simulink model "DETM"  (R2018b)
settings: Solver=ode3  StartTime=0.0  StopTime=55  FixedStep=0.0008  RelTol=1e-3
settings Model: Creator=SURFACE  LastModifiedBy=SURFACE

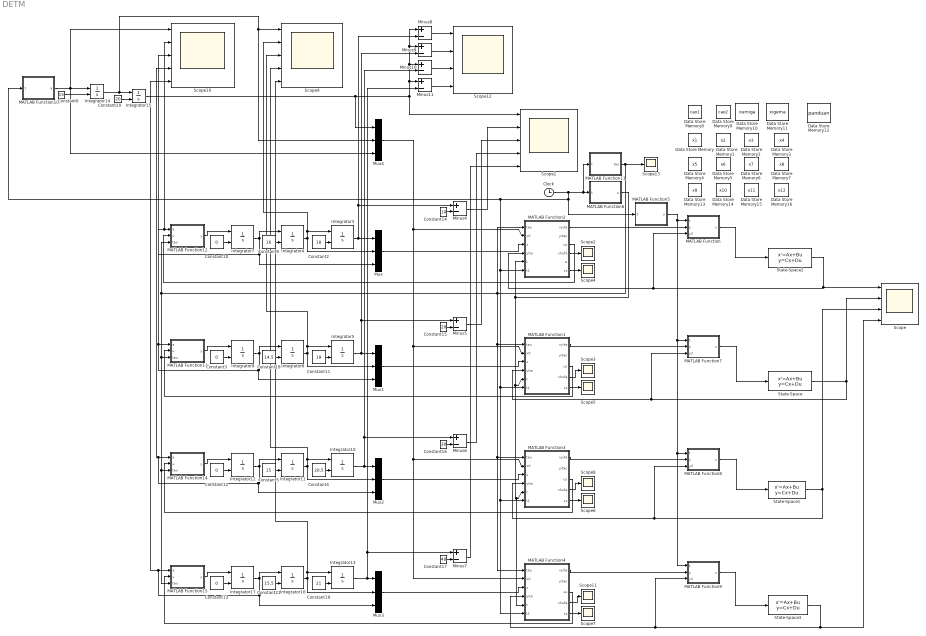
== system DETM ==
  Clock : Clock
  Constant{3,10,12..13} (4 alike) : Constant  Value=0
  Constant11 : Constant  Value=19
  Constant14 : Constant  Value=10
  Constant15 : Constant  Value=20
  Constant16 : Constant  Value=30
  Constant17 : Constant  Value=40
  Constant18 : Constant  Value=14.5
  Constant19 : Constant  Value=21
  Constant2 : Constant  Value=18
  Constant20 : Constant  Value=20
  Constant21 : Constant  Value=15.5
  Constant4 : Constant  Value=20.5
  Constant5 : Constant  Value=15
  Constant6 : Constant  Value=15
  Constant9 : Constant  Value=16
  Data Store Memory : DataStoreMemory  DataStoreName=x1  ReadBeforeWriteMsg=warning  WriteAfterWriteMsg=warning  WriteAfterReadMsg=warning  InitialValue=[18;16;0]  ShowAdditionalParam=off  OutDataTypeStr=double  Dimensions=3
  Data Store Memory1 : DataStoreMemory  DataStoreName=x2  ReadBeforeWriteMsg=warning  WriteAfterWriteMsg=warning  WriteAfterReadMsg=warning  InitialValue=[19;14.5;0]  ShowAdditionalParam=off  OutDataTypeStr=double  Dimensions=3
  Data Store Memory10 : DataStoreMemory  DataStoreName=oumiga  ReadBeforeWriteMsg=warning  WriteAfterWriteMsg=warning  WriteAfterReadMsg=warning  InitialValue=0.5  ShowAdditionalParam=off  OutDataTypeStr=double  Dimensions=1
  Data Store Memory11 : DataStoreMemory  DataStoreName=xigema  ReadBeforeWriteMsg=warning  WriteAfterWriteMsg=warning  WriteAfterReadMsg=warning  InitialValue=3  ShowAdditionalParam=off  OutDataTypeStr=double  Dimensions=1
  Data Store Memory12 : DataStoreMemory  DataStoreName=panduan  ReadBeforeWriteMsg=warning  WriteAfterWriteMsg=warning  WriteAfterReadMsg=warning  InitialValue=1  ShowAdditionalParam=off  OutDataTypeStr=double  Dimensions=1
  Data Store Memory13 : DataStoreMemory  DataStoreName=x9  ReadBeforeWriteMsg=warning  WriteAfterWriteMsg=warning  WriteAfterReadMsg=warning  InitialValue=1  ShowAdditionalParam=off  OutDataTypeStr=double  Dimensions=1
  Data Store Memory14 : DataStoreMemory  DataStoreName=x10  ReadBeforeWriteMsg=warning  WriteAfterWriteMsg=warning  WriteAfterReadMsg=warning  InitialValue=1  ShowAdditionalParam=off  OutDataTypeStr=double  Dimensions=1
  Data Store Memory15 : DataStoreMemory  DataStoreName=x11  ReadBeforeWriteMsg=warning  WriteAfterWriteMsg=warning  WriteAfterReadMsg=warning  InitialValue=1  ShowAdditionalParam=off  OutDataTypeStr=double  Dimensions=1
  Data Store Memory16 : DataStoreMemory  DataStoreName=x12  ReadBeforeWriteMsg=warning  WriteAfterWriteMsg=warning  WriteAfterReadMsg=warning  InitialValue=1  ShowAdditionalParam=off  OutDataTypeStr=double  Dimensions=1
  Data Store Memory2 : DataStoreMemory  DataStoreName=x3  ReadBeforeWriteMsg=warning  WriteAfterWriteMsg=warning  WriteAfterReadMsg=warning  InitialValue=[20.5;15;0]  ShowAdditionalParam=off  OutDataTypeStr=double  Dimensions=3
  Data Store Memory3 : DataStoreMemory  DataStoreName=x4  ReadBeforeWriteMsg=warning  WriteAfterWriteMsg=warning  WriteAfterReadMsg=warning  InitialValue=[21;15.5;0]  ShowAdditionalParam=off  OutDataTypeStr=double  Dimensions=3
  Data Store Memory4 : DataStoreMemory  DataStoreName=x5  ReadBeforeWriteMsg=warning  WriteAfterWriteMsg=warning  WriteAfterReadMsg=warning  ShowAdditionalParam=off  OutDataTypeStr=double  Dimensions=1
  Data Store Memory5 : DataStoreMemory  DataStoreName=x6  ReadBeforeWriteMsg=warning  WriteAfterWriteMsg=warning  WriteAfterReadMsg=warning  ShowAdditionalParam=off  OutDataTypeStr=double  Dimensions=1
  Data Store Memory6 : DataStoreMemory  DataStoreName=x7  ReadBeforeWriteMsg=warning  WriteAfterWriteMsg=warning  WriteAfterReadMsg=warning  ShowAdditionalParam=off  OutDataTypeStr=double  Dimensions=1
  Data Store Memory7 : DataStoreMemory  DataStoreName=x8  ReadBeforeWriteMsg=warning  WriteAfterWriteMsg=warning  WriteAfterReadMsg=warning  ShowAdditionalParam=off  OutDataTypeStr=double  Dimensions=1
  Data Store Memory8 : DataStoreMemory  DataStoreName=cao1  ReadBeforeWriteMsg=warning  WriteAfterWriteMsg=warning  WriteAfterReadMsg=warning  InitialValue=453.396854125846  ShowAdditionalParam=off  OutDataTypeStr=double  Dimensions=1
  Data Store Memory9 : DataStoreMemory  DataStoreName=cao2  ReadBeforeWriteMsg=warning  WriteAfterWriteMsg=warning  WriteAfterReadMsg=warning  InitialValue=7.91493350690816  ShowAdditionalParam=off  OutDataTypeStr=double  Dimensions=1
  Integrator{3..5,7..17} (14 alike) : Integrator  InitialConditionSource=external
  MATLAB Function : MATLAB Function  TreatAsAtomicUnit=on
  MATLAB Function1 : MATLAB Function  TreatAsAtomicUnit=on
  MATLAB Function10 : MATLAB Function  TreatAsAtomicUnit=on
  MATLAB Function11 : MATLAB Function  TreatAsAtomicUnit=on
  MATLAB Function12 : MATLAB Function  TreatAsAtomicUnit=on
  MATLAB Function13 : MATLAB Function  TreatAsAtomicUnit=on
  MATLAB Function14 : MATLAB Function  TreatAsAtomicUnit=on
  MATLAB Function15 : MATLAB Function  TreatAsAtomicUnit=on
  MATLAB Function2 : MATLAB Function  TreatAsAtomicUnit=on
  MATLAB Function3 : MATLAB Function  TreatAsAtomicUnit=on
  MATLAB Function4 : MATLAB Function  TreatAsAtomicUnit=on
  MATLAB Function5 : MATLAB Function  TreatAsAtomicUnit=on
  MATLAB Function6 : MATLAB Function  TreatAsAtomicUnit=on
  MATLAB Function7 : MATLAB Function  TreatAsAtomicUnit=on
  MATLAB Function8 : MATLAB Function  TreatAsAtomicUnit=on
  MATLAB Function9 : MATLAB Function  TreatAsAtomicUnit=on
  Minus{4..11} (8 alike) : Sum  Inputs=+-
  Mux{,1..4} (5 alike) : Mux  Inputs=3
  Scope : Scope  NumInputPorts=4
  Scope1 : Scope  NumInputPorts=5
  Scope10 : Scope  NumInputPorts=5
  Scope{2..8,11,13} (9 alike) : Scope
  Scope12 : Scope  NumInputPorts=4
  Scope9 : Scope  NumInputPorts=5
  State-Space{,1..3} (4 alike) : StateSpace  A=-0.5  B=-1  D=0  InitialCondition=50
  wires:
  Mux4/1 -> MATLAB Function4/2(x0), MATLAB Function3/2(x0), MATLAB Function1/2(x0), MATLAB Function2/2(x0)
  Mux/1 -> MATLAB Function2/3(x)
  Mux1/1 -> MATLAB Function1/3(x)
  Mux2/1 -> MATLAB Function3/3(x)
  Mux3/1 -> MATLAB Function4/3(x)
  Constant14/1 -> Minus4/2
  Constant15/1 -> Minus5/2
  Constant16/1 -> Minus6/2
  Constant17/1 -> Minus7/2
  Minus4/1 -> Scope1/2
  Minus5/1 -> Scope1/3
  Minus6/1 -> Scope1/4
  Minus7/1 -> Scope1/5
  Minus8/1 -> Scope12/1
  Minus9/1 -> Scope12/2
  Minus10/1 -> Scope12/3
  Minus11/1 -> Scope12/4
  Clock/1 -> MATLAB Function4/6(t1), MATLAB Function3/6(t1), MATLAB Function1/6(t1), MATLAB Function2/6(t1), MATLAB Function10/1(t), MATLAB Function5/1(t), MATLAB Function11/1(t), MATLAB Function6/1(t)
  MATLAB Function6/1(u) -> MATLAB Function2/5(t), MATLAB Function4/5(t), MATLAB Function3/5(t), MATLAB Function1/5(t)
  State-Space/1 -> MATLAB Function7/3(y2), MATLAB Function1/4(yita), Scope/2
  MATLAB Function7/1(u) -> State-Space/1
  State-Space1/1 -> MATLAB Function8/3(y2), MATLAB Function3/4(yita), Scope/3
  MATLAB Function/1(u) -> State-Space2/1
  State-Space2/1 -> MATLAB Function/3(y2), MATLAB Function2/4(yita), Scope/1
  State-Space3/1 -> Scope/4, MATLAB Function4/4(yita), MATLAB Function9/3(y2)
  MATLAB Function2/1(vyita) -> MATLAB Function/2(y)
  MATLAB Function5/1(u) -> MATLAB Function9/1(t), MATLAB Function8/1(t), MATLAB Function7/1(t), MATLAB Function/1(t)
  MATLAB Function8/1(u) -> State-Space1/1
  MATLAB Function9/1(u) -> State-Space3/1
  MATLAB Function1/1(vyita) -> MATLAB Function7/2(y)
  MATLAB Function3/1(vyita) -> MATLAB Function8/2(y)
  MATLAB Function4/1(vyita) -> MATLAB Function9/2(y)
  Integrator14/1 -> Mux4/2, Scope9/1, Integrator15/1
  Constant20/1 -> Integrator15/2
  MATLAB Function10/1(a) -> Scope10/1, Mux4/3, Integrator14/1
  Constant6/1 -> Integrator14/2
  Integrator15/1 -> Mux4/1, Scope1/1, Minus11/1, Minus10/1, Minus8/1, Minus9/1
  MATLAB Function12/1(y) -> Integrator7/1
  Integrator4/1 -> Mux/2, Integrator3/1, Scope9/2
  Integrator7/1 -> Mux/3, Scope10/2, MATLAB Function12/1(a), Integrator4/1
  Constant9/1 -> Integrator4/2
  Constant10/1 -> Integrator7/2
  Constant2/1 -> Integrator3/2
  Integrator3/1 -> Minus4/1, Minus8/2, Mux/1
  MATLAB Function2/3(us) -> MATLAB Function12/2(u)
  Constant11/1 -> Integrator5/2
  Constant3/1 -> Integrator9/2
  Constant18/1 -> Integrator8/2
  Integrator9/1 -> Integrator8/1, Mux1/3, Scope10/3, MATLAB Function13/1(a)
  Integrator8/1 -> Mux1/2, Scope9/3, Integrator5/1
  MATLAB Function13/1(y) -> Integrator9/1
  MATLAB Function14/1(y) -> Integrator12/1
  Integrator11/1 -> Mux2/2, Integrator10/1, Scope9/4
  Integrator12/1 -> Mux2/3, MATLAB Function14/1(a), Scope10/4, Integrator11/1
  Constant5/1 -> Integrator11/2
  Constant12/1 -> Integrator12/2
  Constant4/1 -> Integrator10/2
  Constant19/1 -> Integrator13/2
  Constant13/1 -> Integrator17/2
  Constant21/1 -> Integrator16/2
  Integrator17/1 -> Integrator16/1, Mux3/3, Scope10/5, MATLAB Function15/1(a)
  Integrator16/1 -> Mux3/2, Scope9/5, Integrator13/1
  MATLAB Function15/1(y) -> Integrator17/1
  Integrator5/1 -> Minus5/1, Minus9/2, Mux1/1
  Integrator10/1 -> Minus6/1, Minus10/2, Mux2/1
  Integrator13/1 -> Minus7/1, Minus11/2, Mux3/1
  MATLAB Function1/3(us) -> MATLAB Function13/2(u)
  MATLAB Function3/3(us) -> MATLAB Function14/2(u)
  MATLAB Function4/3(us) -> MATLAB Function15/2(u)
  MATLAB Function11/1(tau) -> Scope13/1, MATLAB Function4/1(tau), MATLAB Function3/1(tau), MATLAB Function1/1(tau), MATLAB Function2/1(tau), MATLAB Function15/3(tau), MATLAB Function14/3(tau), MATLAB Function13/3(tau), MATLAB Function12/3(tau)
  MATLAB Function2/6(cs) -> Scope4/1
  MATLAB Function2/4(chufa) -> Scope2/1
  MATLAB Function1/4(chufa) -> Scope3/1
  MATLAB Function1/5(cs) -> Scope5/1
  MATLAB Function3/5(cs) -> Scope6/1
  MATLAB Function4/5(cs) -> Scope7/1
  MATLAB Function3/4(chufa) -> Scope8/1
  MATLAB Function4/4(chufa) -> Scope11/1

== matlab function DETM/MATLAB Function1 ==
  settings: updateMethod=DISCRETE
  data: tau input; x0 input; x input; vyita output; yita input; yitac output; us output; x1 data_store_memory; x2 data_store_memory; x3 data_store_memory; x4 data_store_memory; x6 data_store_memory; chufa output; cao1 data_store_memory; cao2 data_store_memory; xigema data_store_memory; oumiga data_store_memory; t input; t1 input; x10 data_store_memory; cs output
function [vyita,yitac,us,chufa,cs]  =fcn(tau,x0,x,yita,t,t1)
global x1;
global x2;
global x3;
global x4;
global x6;
global x10;
global cao1;
global cao2;
global xigema;
global oumiga;
x0hat=[];
H=[1 0 0 0;
   0 1 0 0;
   0 0 0 0;
   0 0 0 0];
L=[1 -1 0 0;
  -1 2 -1 0;
  -1 -1 3 -1;
   0 -1 -1 2];
q=[0 0 0 0;
   0 0 0 0;
   0 0 0 0];%q更新
B=[0 0 1/0.34];%为了方便转置了一下
P=[ 2.2028   -1.6797    1.4243;
   -1.6797    1.8580   -2.7082;
    1.4243   -2.7082    6.4228];
o=[x1 x2 x3 x4];
for i=1:4%计算q值与输入u
    q(:,i)=q(:,i)+H(i,i)*(o(:,i)-x0);
    for k=1:4
    q(:,i)=q(:,i)+L(i,k)*(o(:,k));
    end
end
u=-B*inv(P)*q*t;%控制输入
vyita=oumiga*(cao1*(norm(x2-x))^2-cao2*(norm(q(:,2)))^2);
yitac=xigema*(cao1*(norm(x2-x))^2-cao2*(norm(q(:,2)))^2)*t;
if yitac>=yita
x10=x10+1;
x2=x;
chufa=t1-x6;
x6=t1;
else
chufa=0;
end
coder.extrinsic('GuvDETM');
x2=GuvDETM(x2,1/tau);
us=u(1,2);%要改的
cs=x10;

== matlab function DETM/MATLAB Function3 ==
  settings: updateMethod=DISCRETE
  data: tau input; x0 input; x input; vyita output; yita input; yitac output; us output; x1 data_store_memory; x2 data_store_memory; x3 data_store_memory; x4 data_store_memory; chufa output; x7 data_store_memory; cao1 data_store_memory; cao2 data_store_memory; xigema data_store_memory; oumiga data_store_memory; t input; t1 input; x11 data_store_memory; cs output
function [vyita,yitac,us,chufa,cs]  =fcn(tau,x0,x,yita,t,t1)
global x1;
global x2;
global x3;
global x4;
global x7;
global x11;
global cao1;
global cao2;
global xigema;
global oumiga;
H=[1 0 0 0;
   0 1 0 0;
   0 0 0 0;
   0 0 0 0];
L=[1 -1 0 0;
  -1 2 -1 0;
  -1 -1 3 -1;
   0 -1 -1 2];
q=[0 0 0 0;
   0 0 0 0;
   0 0 0 0];%q更新
B=[0 0 1/0.34];%为了方便转置了一下
P=[ 2.2028   -1.6797    1.4243;
   -1.6797    1.8580   -2.7082;
    1.4243   -2.7082    6.4228];
o=[x1 x2 x3 x4];
for i=1:4%计算q值与输入u
    q(:,i)=q(:,i)+H(i,i)*(o(:,i)-x0);
    for k=1:4
    q(:,i)=q(:,i)+L(i,k)*(o(:,k));
    end
end
u=-B*inv(P)*q*t;%控制输入
vyita=oumiga*(cao1*(norm(x3-x))^2-cao2*(norm(q(:,3)))^2);
yitac=xigema*(cao1*(norm(x3-x))^2-cao2*(norm(q(:,3)))^2)*t;
if yitac>=yita
x11=x11+1;
x3=x;
chufa=t1-x7;
x7=t1;
else
chufa=0;
end
coder.extrinsic('GuvDETM');
x3=GuvDETM(x3,1/tau);
us=u(1,3);%要改的
cs=x11;

== matlab function DETM/MATLAB Function2 ==
  settings: updateMethod=DISCRETE
  data: tau input; x0 input; x input; vyita output; yita input; yitac output; us output; x1 data_store_memory; x2 data_store_memory; x3 data_store_memory; x4 data_store_memory; x5 data_store_memory; chufa output; cao1 data_store_memory; cao2 data_store_memory; xigema data_store_memory; oumiga data_store_memory; t input; e output; t1 input; x9 data_store_memory; cs output
function [vyita,yitac,us,chufa,e,cs]  =fcn(tau,x0,x,yita,t,t1)
global x1;
global x2;
global x3;
global x4;
global x5;
global x9;
global cao1;
global cao2;
global xigema;
global oumiga;
e=0;
H=[1 0 0 0;
   0 1 0 0;
   0 0 0 0;
   0 0 0 0];
L=[1 -1 0 0;
  -1 2 -1 0;
  -1 -1 3 -1;
   0 -1 -1 2];
q=[0 0 0 0;
   0 0 0 0;
   0 0 0 0];%q更新
B=[0 0 1/0.34];%为了方便转置了一下
P=[ 2.2028   -1.6797    1.4243;
   -1.6797    1.8580   -2.7082;
    1.4243   -2.7082    6.4228];
o=[x1 x2 x3 x4];
for i=1:4%计算q值与输入u
    q(:,i)=q(:,i)+H(i,i)*(o(:,i)-x0);
    for k=1:4
    q(:,i)=q(:,i)+L(i,k)*(o(:,k));
    end
end
u=-B*inv(P)*q*t;%控制输入
vyita=oumiga*(cao1*(norm(x1-x)^2)-cao2*(norm(q(:,1)))^2);
yitac=xigema*(cao1*(norm(x1-x)^2)-cao2*(norm(q(:,1)))^2)*t;
if yitac>=yita
x9=x9+1;
x1=x;
chufa=t1-x5;
x5=t1;
else
chufa=0;
end
coder.extrinsic('GuvDETM');
x1=GuvDETM(x1,1/tau);
us=u(1,1);%要改的
e=cao1*norm(x1-x);
cs=x9;

== matlab function DETM/MATLAB Function4 ==
  settings: updateMethod=DISCRETE
  data: tau input; x0 input; x input; vyita output; yita input; yitac output; us output; x1 data_store_memory; x2 data_store_memory; x3 data_store_memory; x4 data_store_memory; x8 data_store_memory; chufa output; cao1 data_store_memory; cao2 data_store_memory; xigema data_store_memory; oumiga data_store_memory; t input; t1 input; x12 data_store_memory; cs output
function [vyita,yitac,us,chufa,cs]  =fcn(tau,x0,x,yita,t,t1)
global x1;
global x2;
global x3;
global x4;
global x8;
global x12;
global cao1;
global cao2;
global xigema;
global oumiga;
H=[1 0 0 0;
   0 1 0 0;
   0 0 0 0;
   0 0 0 0];
L=[1 -1 0 0;
  -1 2 -1 0;
  -1 -1 3 -1;
   0 -1 -1 2];
q=[0 0 0 0;
   0 0 0 0;
   0 0 0 0];%q更新
B=[0 0 1/0.34];%为了方便转置了一下
P=[ 2.2028   -1.6797    1.4243;
   -1.6797    1.8580   -2.7082;
    1.4243   -2.7082    6.4228];
o=[x1 x2 x3 x4];
for i=1:4%计算q值与输入u
    q(:,i)=q(:,i)+H(i,i)*(o(:,i)-x0);
    for k=1:4
    q(:,i)=q(:,i)+L(i,k)*(o(:,k));
    end
end
u=-B*inv(P)*q*t;%控制输入
vyita=oumiga*(cao1*(norm(x4-x))^2-cao2*(norm(q(:,4)))^2);
yitac=xigema*(cao1*(norm(x4-x))^2-cao2*(norm(q(:,4)))^2)*t;
if yitac>=yita
x12=x12+1;
x4=x;
chufa=t1-x8;
x8=t1;
else
chufa=0;
end
coder.extrinsic('GuvDETM');
x4=GuvDETM(x4,1/tau);
us=u(1,4);%要改的
cs=x12;

== matlab function DETM/MATLAB Function5 ==
  data: t input; u output

function u  = fcn(t)
u=1;
if t<=3
    u=1;
elseif t<=5.02
    u=0;
elseif t<=10.5
    u=1;
elseif t<=12.02
    u=0;
elseif t<=13.5
    u=1;
elseif t<=14.02
    u=0;
elseif t<=25
    u=1;
elseif t<=26.52
    u=0;
elseif t<=36
    u=1;
elseif t<=37.02
    u=0;
elseif t<=38
    u=1;
elseif t<=39.52
    u=0;
elseif t<=52
    u=1; 
elseif t<=54.02
    u=0;
elseif t<=65
    u=1;
end

== matlab function DETM/MATLAB Function6 ==
  data: t input; u output

function u  = fcn(t)
u=1;
if t<=3
    u=1;
elseif t<=5
    u=0;
elseif t<=10.5
    u=1;
elseif t<=12
    u=0;
elseif t<=13.5
    u=1;
elseif t<=14
    u=0;
elseif t<=25
    u=1;
elseif t<=26.5
    u=0;
elseif t<=36
    u=1;
elseif t<=37
    u=0;
elseif t<=38
    u=1;
elseif t<=39.5
    u=0;
elseif t<=52
    u=1; 
elseif t<=54
    u=0;
elseif t<=55
    u=1;
end

== matlab function DETM/MATLAB Function ==
  data: t input; u output; y input; y2 input

function u  = fcn(t,y,y2)
u=1;
if t==1
    u=y*t;
elseif t==0
    u=-0.5*y2;
end

== matlab function DETM/MATLAB Function7 ==
  data: t input; u output; y input; y2 input

function u  = fcn(t,y,y2)
u=1;
if t==1
    u=y*t;
elseif t==0
    u=-0.5*y2;
end

== matlab function DETM/MATLAB Function8 ==
  data: t input; u output; y input; y2 input

function u  = fcn(t,y,y2)
u=1;
if t==1
    u=y*t;
elseif t==0
    u=-0.5*y2;
end

== matlab function DETM/MATLAB Function9 ==
  data: t input; u output; y input; y2 input

function u  = fcn(t,y,y2)
u=1;
if t==1
    u=y*t;
elseif t==0
    u=-0.5*y2;
end

== matlab function DETM/MATLAB Function10 ==
  data: t input; a output
function a   = fcn(t)
a=0;
if t<=10
 a=0;
elseif t<=15
a=2;   
elseif t<=35
a=0;    
elseif t<=40
a=-2;   
elseif t<=55
a=0;   
end

== matlab function DETM/MATLAB Function11 ==
  data: t input; tau output

function tau  = fcn(t)
tau=0.34;
if t<=20
    tau=0.34;
elseif t<=35
    tau=0.34+0.48/15*(t-20);
elseif t<=55
    tau=0.82;
end

== matlab function DETM/MATLAB Function12 ==
  data: a input; u input; y output; tau input
function y = fcn(a,u,tau)
y=-1/tau*(a-u);

== matlab function DETM/MATLAB Function13 ==
  data: a input; u input; y output; tau input
function y = fcn(a,u,tau)
y=-1/tau*(a-u);

== matlab function DETM/MATLAB Function14 ==
  data: a input; u input; y output; tau input
function y = fcn(a,u,tau)
y=-1/tau*(a-u);

== matlab function DETM/MATLAB Function15 ==
  data: a input; u input; y output; tau input
function y = fcn(a,u,tau)
y=-1/tau*(a-u);
